simulink model "Par62"  (R2018a)
settings: Solver=FixedStepAuto  StartTime=0.0  StopTime=100  FixedStep=0.1  RelTol=1e-3
settings Model: Creator=wangluo  LastModifiedBy=wangluo

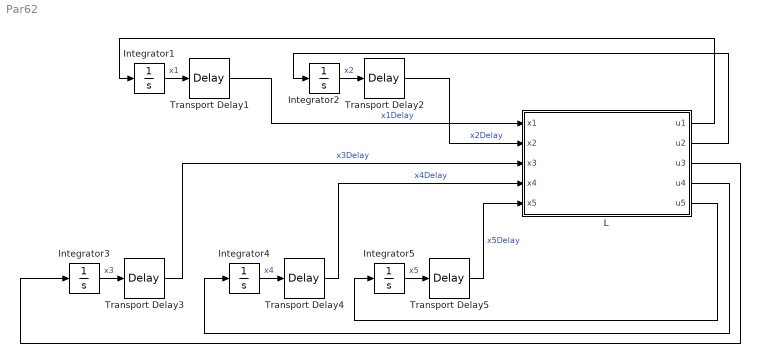
== system Par62 ==
  Integrator1 : Integrator  InitialCondition=8.9
  Integrator2 : Integrator  InitialCondition=3.5
  Integrator3 : Integrator  InitialCondition=5.5
  Integrator4 : Integrator  InitialCondition=4.5
  Integrator5 : Integrator  InitialCondition=2.7
  L : Subsystem
  Transport Delay1 : TransportDelay  DelayTime=0.2
  Transport Delay2 : TransportDelay  DelayTime=0.1
  Transport Delay3 : TransportDelay  DelayTime=0.05
  Transport Delay5 : TransportDelay  DelayTime=0.2
  Transport Delay4 : TransportDelay  DelayTime=0.06
  wires:
  Integrator1/1 -> Transport Delay1/1  "x1"
  Integrator2/1 -> Transport Delay2/1  "x2"
  Integrator3/1 -> Transport Delay3/1  "x3"
  L/2(u2) -> Integrator2/1
  L/1(u1) -> Integrator1/1
  L/3(u3) -> Integrator3/1
  L/4(u4) -> Integrator4/1
  L/5(u5) -> Integrator5/1
  Transport Delay4/1 -> L/4(x4)  "x4Delay"
  Transport Delay3/1 -> L/3(x3)  "x3Delay"
  Transport Delay5/1 -> L/5(x5)  "x5Delay"
  Transport Delay1/1 -> L/1(x1)  "x1Delay"
  Transport Delay2/1 -> L/2(x2)  "x2Delay"
  Integrator4/1 -> Transport Delay4/1  "x4"
  Integrator5/1 -> Transport Delay5/1  "x5"

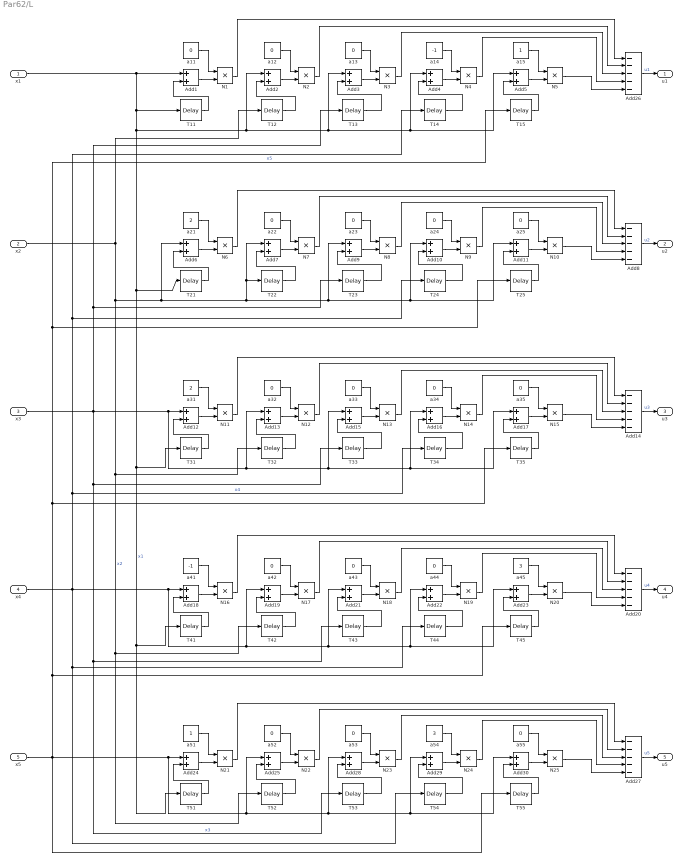
== system Par62/L ==
  x1 : Inport
  x2 : Inport  Port=2
  x3 : Inport  Port=3
  x4 : Inport  Port=4
  x5 : Inport  Port=5
  Add{1..7,9..13,15..19,21..25,28..30} (25 alike) : Sum
  Add{8,14,20,26..27} (5 alike) : Sum  Inputs=-----
  N{1..25} (25 alike) : Product
  T{11..15,21..25,31..35,41..45,51..55} (25 alike) : TransportDelay  DelayTime=0.3
  a{11..13,22..25,32..35,42..44,52..53,55} (17 alike) : Constant  Value=0
  a14 : Constant  Value=-1
  a15 : Constant
  a21 : Constant  Value=2
  a31 : Constant  Value=2
  a41 : Constant  Value=-1
  a45 : Constant  Value=3
  a51 : Constant
  a54 : Constant  Value=3
  u1 : Outport
  u2 : Outport  Port=2
  u3 : Outport  Port=3
  u4 : Outport  Port=4
  u5 : Outport  Port=5
  wires:
  Add26/1 -> u1/1  "u1"
  Add8/1 -> u2/1  "u2"
  T11/1 -> Add1/2
  Add1/1 -> N1/2
  a11/1 -> N1/1
  T12/1 -> Add2/2
  Add2/1 -> N2/2
  a12/1 -> N2/1
  T13/1 -> Add3/2
  Add3/1 -> N3/2
  a13/1 -> N3/1
  T14/1 -> Add4/2
  Add4/1 -> N4/2
  a14/1 -> N4/1
  T15/1 -> Add5/2
  Add5/1 -> N5/2
  a15/1 -> N5/1
  N5/1 -> Add26/5
  N4/1 -> Add26/4
  N3/1 -> Add26/3
  N2/1 -> Add26/2
  N1/1 -> Add26/1
  x1/1 -> Add1/1, T11/1, Add2/1, Add3/1, Add4/1, Add5/1, T21/1, T31/1, T51/1, T41/1  "x1"
  a23/1 -> N8/1
  a24/1 -> N9/1
  Add10/1 -> N9/2
  T22/1 -> Add7/2
  a22/1 -> N7/1
  Add7/1 -> N7/2
  Add9/1 -> N8/2
  T24/1 -> Add10/2
  N8/1 -> Add8/3
  x2/1 -> Add7/1, T22/1, Add9/1, Add10/1, Add11/1, Add6/1, T32/1, T42/1, T52/1, T12/1  "x2"
  T21/1 -> Add6/2
  a25/1 -> N10/1
  a21/1 -> N6/1
  Add6/1 -> N6/2
  N7/1 -> Add8/2
  T23/1 -> Add9/2
  T25/1 -> Add11/2
  Add11/1 -> N10/2
  N10/1 -> Add8/5
  N6/1 -> Add8/1
  N9/1 -> Add8/4
  a33/1 -> N13/1
  a34/1 -> N14/1
  Add16/1 -> N14/2
  T32/1 -> Add13/2
  a32/1 -> N12/1
  Add13/1 -> N12/2
  Add14/1 -> u3/1  "u3"
  Add15/1 -> N13/2
  T34/1 -> Add16/2
  N13/1 -> Add14/3
  x3/1 -> T33/1, T53/1, T43/1, T23/1, T13/1, Add13/1, Add15/1, Add16/1, Add17/1, Add12/1  "x3"
  T31/1 -> Add12/2
  a35/1 -> N15/1
  a31/1 -> N11/1
  Add12/1 -> N11/2
  N12/1 -> Add14/2
  T33/1 -> Add15/2
  T35/1 -> Add17/2
  Add17/1 -> N15/2
  N15/1 -> Add14/5
  N11/1 -> Add14/1
  N14/1 -> Add14/4
  a43/1 -> N18/1
  a44/1 -> N19/1
  Add22/1 -> N19/2
  T42/1 -> Add19/2
  a42/1 -> N17/1
  Add19/1 -> N17/2
  Add21/1 -> N18/2
  T44/1 -> Add22/2
  N18/1 -> Add20/3
  x4/1 -> T44/1, T54/1, Add19/1, Add21/1, Add22/1, Add23/1, Add18/1, T24/1, T14/1, T34/1  "x4"
  T41/1 -> Add18/2
  a45/1 -> N20/1
  a41/1 -> N16/1
  Add18/1 -> N16/2
  N17/1 -> Add20/2
  T43/1 -> Add21/2
  T45/1 -> Add23/2
  Add23/1 -> N20/2
  N20/1 -> Add20/5
  N16/1 -> Add20/1
  N19/1 -> Add20/4
  a53/1 -> N23/1
  a54/1 -> N24/1
  Add29/1 -> N24/2
  T52/1 -> Add25/2
  a52/1 -> N22/1
  Add25/1 -> N22/2
  Add27/1 -> u5/1  "u5"
  Add28/1 -> N23/2
  T54/1 -> Add29/2
  N23/1 -> Add27/3
  x5/1 -> Add25/1, Add28/1, Add29/1, Add30/1, Add24/1, T55/1, T45/1, T35/1, T25/1, T15/1  "x5"
  T51/1 -> Add24/2
  a55/1 -> N25/1
  a51/1 -> N21/1
  Add24/1 -> N21/2
  N22/1 -> Add27/2
  T53/1 -> Add28/2
  T55/1 -> Add30/2
  Add30/1 -> N25/2
  N25/1 -> Add27/5
  N21/1 -> Add27/1
  N24/1 -> Add27/4
  Add20/1 -> u4/1  "u4"
